simulink model "DoAero_2008a"  (Simulink 7.1)
settings: Solver=ode3  StartTime=0.0  StopTime=100  FixedStep=0.01  RelTol=1e-3
settings Model: Creator=abdelrazzak.merheb  LastModifiedBy=flying
settings OptimizationCC: InitFltsAndDblsToZero=off
settings DebuggingCC: StrictBusMsg=ErrorLevel1
settings CodeAppCC: CustomSymbolStrType=$N$R$M_T
settings GRTTargetCC: TargetFunctionLibrary=C89/C90 (ANSI)  CPPClassGenCompliant=off

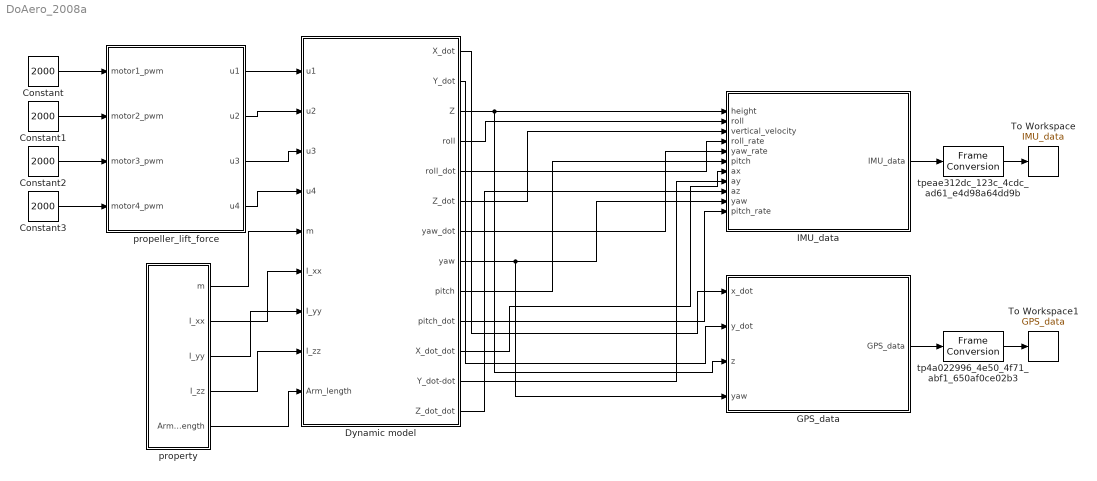
== system DoAero_2008a ==
  Constant{,1..3} (4 alike) : Constant  Value=2000
  Dynamic model : Subsystem
  GPS_data : Subsystem
  IMU_data : Subsystem
  To Workspace : ToWorkspace  VariableName=IMU_data  SampleTime=-1
  To Workspace1 : ToWorkspace  VariableName=GPS_data  SampleTime=-1
  propeller_lift_force : Stateflow chart  TreatAsAtomicUnit=on
      settings: PermitHierarchicalResolution=ParametersOnly
  "property " : Subsystem
  tp4a022996_4e50_4f71_abf1_650af0ce02b3 : FrameConversion
  tpeae312dc_123c_4cdc_ad61_e4d98a64dd9b : FrameConversion
  wires:
  Dynamic model/9(pitch) -> IMU_data/6(pitch)
  Dynamic model/3(Z) -> GPS_data/3(z), IMU_data/1(height)
  Dynamic model/4(roll) -> IMU_data/2(roll)
  Dynamic model/6(Z_dot) -> IMU_data/3(vertical_velocity)
  Dynamic model/5(roll_dot) -> IMU_data/4(roll_rate)
  Dynamic model/10(pitch_dot) -> IMU_data/11(pitch_rate)
  Dynamic model/7(yaw_dot) -> IMU_data/5(yaw_rate)
  Dynamic model/8(yaw) -> GPS_data/4(yaw), IMU_data/10(yaw)
  Dynamic model/11(X_dot_dot) -> IMU_data/7(ax)
  Dynamic model/12(Y_dot-dot) -> IMU_data/8(ay)
  Dynamic model/13(Z_dot_dot) -> IMU_data/9(az)
  "property "/5("Arm_length ") -> Dynamic model/9(Arm_length)
  "property "/4(I_zz) -> Dynamic model/8(I_zz)
  "property "/3(I_yy) -> Dynamic model/7(I_yy)
  "property "/2(I_xx) -> Dynamic model/6(I_xx)
  "property "/1(m) -> Dynamic model/5(m)
  propeller_lift_force/2(u2) -> Dynamic model/2(u2)
  propeller_lift_force/3(u3) -> Dynamic model/3(u3)
  propeller_lift_force/1(u1) -> Dynamic model/1(u1)
  propeller_lift_force/4(u4) -> Dynamic model/4(u4)
  Dynamic model/1("X_dot ") -> GPS_data/1(x_dot)
  Dynamic model/2(Y_dot) -> GPS_data/2(y_dot)
  Constant/1 -> propeller_lift_force/1(motor1_pwm)
  Constant1/1 -> propeller_lift_force/2(motor2_pwm)
  Constant2/1 -> propeller_lift_force/3(motor3_pwm)
  Constant3/1 -> propeller_lift_force/4(motor4_pwm)
  IMU_data/1(IMU_data) -> tpeae312dc_123c_4cdc_ad61_e4d98a64dd9b/1
  tpeae312dc_123c_4cdc_ad61_e4d98a64dd9b/1 -> To Workspace/1
  GPS_data/1(GPS_data) -> tp4a022996_4e50_4f71_abf1_650af0ce02b3/1
  tp4a022996_4e50_4f71_abf1_650af0ce02b3/1 -> To Workspace1/1

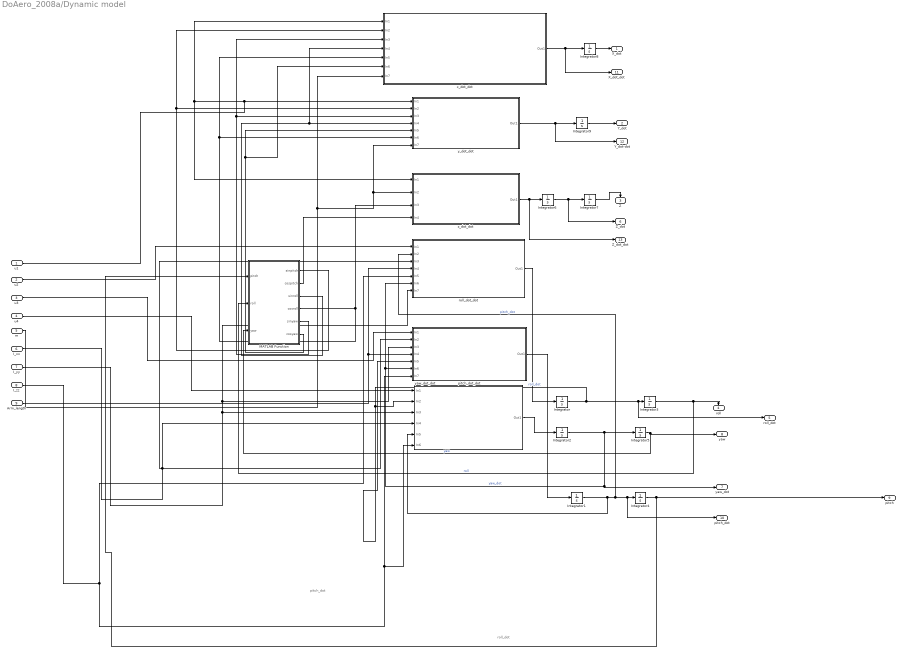
== system DoAero_2008a/Dynamic model ==
  note: pitch_dot
  note: roll_dot
  u1 : Inport
  u2 : Inport  Port=2
  u3 : Inport  Port=3
  u4 : Inport  Port=4
  m : Inport  Port=5
  I_xx : Inport  Port=6
  I_yy : Inport  Port=7
  I_zz : Inport  Port=8
  Arm_length : Inport  Port=9
  Integrator{,1..9} (10 alike) : Integrator
  MATLAB Function : Stateflow chart  TreatAsAtomicUnit=on
      settings: PermitHierarchicalResolution=ParametersOnly
  pitch_dot_dot : Subsystem
  roll_dot_dot : Subsystem
  x_dot_dot : Subsystem
  y_dot_dot : Subsystem
  yaw_dot_dot : Subsystem
  z_dot_dot : Subsystem
  "X_dot " : Outport
  Y_dot : Outport  Port=2
  Z : Outport  Orientation=down  Port=3
  roll : Outport  Orientation=down  Port=4
  roll_dot : Outport  Port=5
  Z_dot : Outport  Port=6
  yaw_dot : Outport  Port=7
  yaw : Outport  Port=8
  pitch : Outport  Port=9
  pitch_dot : Outport  Port=10
  X_dot_dot : Outport  Port=11
  Y_dot-dot : Outport  Port=12
  Z_dot_dot : Outport  Port=13
  wires:
  x_dot_dot/1(Out1) -> X_dot_dot/1, Integrator8/1
  Integrator6/1 -> Integrator7/1, Z_dot/1
  u4/1 -> yaw_dot_dot/1(In1)
  MATLAB Function/6(cosyaw) -> x_dot_dot/6(In6), y_dot_dot/5(In5)
  MATLAB Function/3(sinroll) -> x_dot_dot/4(In4), y_dot_dot/4(In4)
  MATLAB Function/4(cosroll) -> x_dot_dot/5(In5), y_dot_dot/6(In6), z_dot_dot/3(In3)
  MATLAB Function/1(sinpitch) -> x_dot_dot/2(In2), y_dot_dot/2(In2)
  m/1 -> x_dot_dot/7(In7), z_dot_dot/2(In2), y_dot_dot/7(In7)
  MATLAB Function/5(sinyaw) -> x_dot_dot/3(In3), y_dot_dot/3(In3)
  u1/1 -> y_dot_dot/1(In1), x_dot_dot/1(In1), z_dot_dot/1(In1)
  I_xx/1 -> yaw_dot_dot/4(In4), roll_dot_dot/3(In3), pitch_dot_dot/2(In2)
  I_yy/1 -> yaw_dot_dot/3(In3), roll_dot_dot/7(In7), pitch_dot_dot/3(In3)
  I_zz/1 -> roll_dot_dot/5(In5), yaw_dot_dot/6(In6), pitch_dot_dot/7(In7)
  Integrator3/1 -> roll/1, MATLAB Function/2(roll)  "roll"
  Integrator1/1 -> yaw_dot_dot/5(In5), roll_dot_dot/2(In2), pitch_dot/1, Integrator4/1  "pitch_dot"
  Integrator2/1 -> roll_dot_dot/6(In6), pitch_dot_dot/6(In6), yaw_dot/1, Integrator5/1  "yaw_dot"
  Integrator/1 -> pitch_dot_dot/5(In5), yaw_dot_dot/2(In2), roll_dot/1, Integrator3/1  "roll_dot"
  Integrator8/1 -> "X_dot "/1
  Integrator9/1 -> Y_dot/1
  Integrator5/1 -> MATLAB Function/3(yaw), yaw/1  "yaw"
  z_dot_dot/1(Out1) -> Z_dot_dot/1, Integrator6/1
  roll_dot_dot/1(Out1) -> Integrator/1
  pitch_dot_dot/1(Out1) -> Integrator1/1
  MATLAB Function/2(cospitch) -> z_dot_dot/4(In4)
  u2/1 -> roll_dot_dot/1(In1)
  Arm_length/1 -> roll_dot_dot/4(In4), pitch_dot_dot/4(In4)
  u3/1 -> pitch_dot_dot/1(In1)
  y_dot_dot/1(Out1) -> Y_dot-dot/1, Integrator9/1
  Integrator4/1 -> pitch/1, MATLAB Function/1(pitch)
  Integrator7/1 -> Z/1
  yaw_dot_dot/1(Out1) -> Integrator2/1

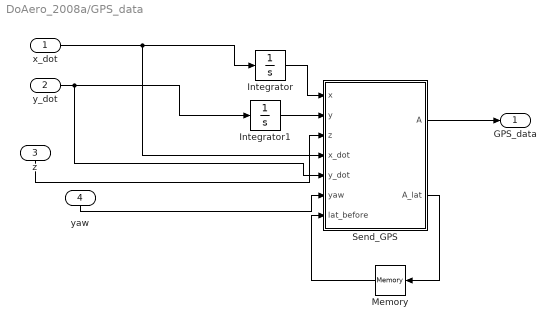
== system DoAero_2008a/GPS_data ==
  x_dot : Inport
  y_dot : Inport  Port=2
  z : Inport  Orientation=down  Port=3
  yaw : Inport  Orientation=down  Port=4
  Integrator : Integrator
  Integrator1 : Integrator
  Memory : Memory  Orientation=left  X0=30
  Send_GPS : Stateflow chart  TreatAsAtomicUnit=on
      settings: PermitHierarchicalResolution=ParametersOnly
  GPS_data : Outport
  wires:
  Integrator/1 -> Send_GPS/1(x)
  Integrator1/1 -> Send_GPS/2(y)
  Send_GPS/1(A) -> GPS_data/1
  yaw/1 -> Send_GPS/6(yaw)
  z/1 -> Send_GPS/3(z)
  Memory/1 -> Send_GPS/7(lat_before)
  Send_GPS/2(A_lat) -> Memory/1
  x_dot/1 -> Integrator/1, Send_GPS/4(x_dot)
  y_dot/1 -> Send_GPS/5(y_dot), Integrator1/1

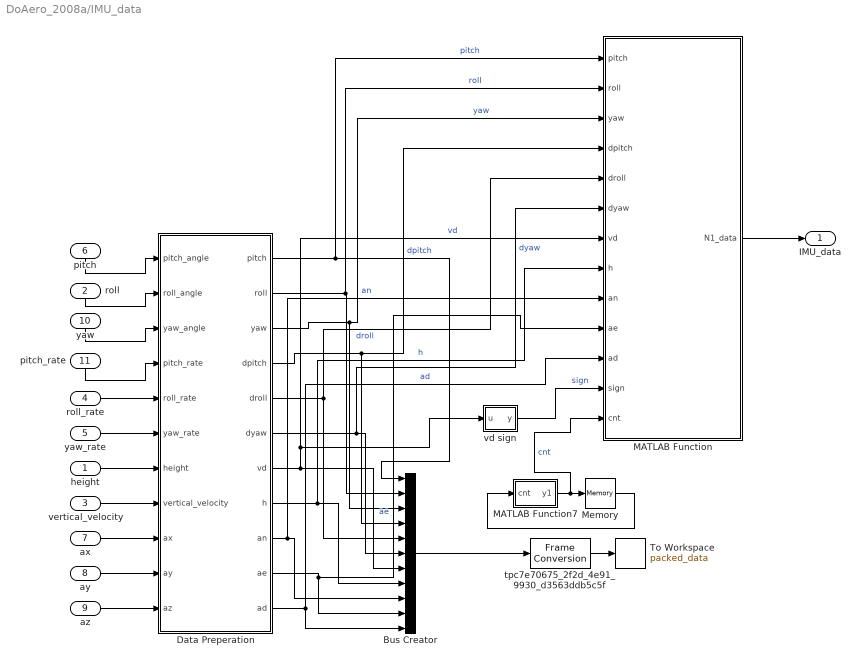
== system DoAero_2008a/IMU_data ==
  height : Inport
  roll : Inport  Orientation=down  Port=2
  vertical_velocity : Inport  Port=3
  roll_rate : Inport  Port=4
  yaw_rate : Inport  Port=5
  pitch : Inport  Orientation=down  Port=6
  ax : Inport  Port=7
  ay : Inport  Port=8
  az : Inport  Port=9
  yaw : Inport  Orientation=down  Port=10
  pitch_rate : Inport  Orientation=down  Port=11
  Bus Creator : BusCreator  Inputs=11
  Data Preperation : Stateflow chart  TreatAsAtomicUnit=on
      settings: PermitHierarchicalResolution=ParametersOnly
  MATLAB Function : Stateflow chart  TreatAsAtomicUnit=on
      settings: PermitHierarchicalResolution=ParametersOnly
  MATLAB Function7 : Stateflow chart  TreatAsAtomicUnit=on
      settings: PermitHierarchicalResolution=ParametersOnly
  Memory : Memory
  To Workspace : ToWorkspace  VariableName=packed_data  SampleTime=-1
  tpc7e70675_2f2d_4e91_9930_d3563ddb5c5f : FrameConversion
  vd sign : Stateflow chart  TreatAsAtomicUnit=on
      settings: PermitHierarchicalResolution=ParametersOnly
  IMU_data : Outport
  wires:
  Data Preperation/5(droll) -> MATLAB Function/5(droll), Bus Creator/5  "droll"
  Data Preperation/10(ae) -> MATLAB Function/10(ae), Bus Creator/10  "ae"
  ax/1 -> Data Preperation/9(ax)
  Data Preperation/6(dyaw) -> MATLAB Function/6(dyaw), Bus Creator/6  "dyaw"
  Data Preperation/7(vd) -> MATLAB Function/7(vd), vd sign/1(u), Bus Creator/7  "vd"
  Data Preperation/8(h) -> MATLAB Function/8(h), Bus Creator/8  "h"
  Data Preperation/3(yaw) -> MATLAB Function/3(yaw), Bus Creator/3  "yaw"
  Data Preperation/9(an) -> MATLAB Function/9(an), Bus Creator/9  "an"
  Data Preperation/4(dpitch) -> MATLAB Function/4(dpitch), Bus Creator/4  "dpitch"
  vd sign/1(y) -> MATLAB Function/12(sign)  "sign"
  MATLAB Function7/1(y1) -> MATLAB Function/13(cnt), Memory/1  "cnt"
  Data Preperation/2(roll) -> MATLAB Function/2(roll), Bus Creator/2  "roll"
  ay/1 -> Data Preperation/10(ay)
  Data Preperation/11(ad) -> MATLAB Function/11(ad), Bus Creator/11  "ad"
  Data Preperation/1(pitch) -> MATLAB Function/1(pitch), Bus Creator/1  "pitch"
  az/1 -> Data Preperation/11(az)
  Memory/1 -> MATLAB Function7/1(cnt)
  yaw_rate/1 -> Data Preperation/6(yaw_rate)
  height/1 -> Data Preperation/7(height)
  yaw/1 -> Data Preperation/3(yaw_angle)
  pitch/1 -> Data Preperation/1(pitch_angle)
  roll_rate/1 -> Data Preperation/5(roll_rate)
  pitch_rate/1 -> Data Preperation/4(pitch_rate)
  vertical_velocity/1 -> Data Preperation/8(vertical_velocity)
  roll/1 -> Data Preperation/2(roll_angle)
  MATLAB Function/1(N1_data) -> IMU_data/1
  Bus Creator/1 -> tpc7e70675_2f2d_4e91_9930_d3563ddb5c5f/1
  tpc7e70675_2f2d_4e91_9930_d3563ddb5c5f/1 -> To Workspace/1

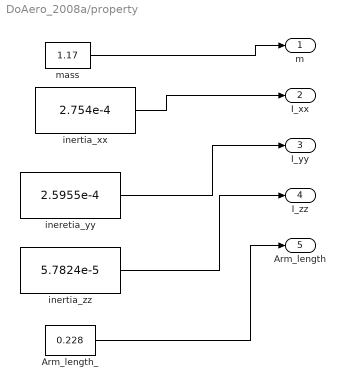
== system DoAero_2008a/property  ==
  Arm_length_ : Constant  Value=0.228
  ineretia_yy : Constant  Value=2.5955e-4
  inertia_xx : Constant  Value=2.754e-4
  inertia_zz : Constant  Value=5.7824e-5
  mass : Constant  Value=1.17
  m : Outport
  I_xx : Outport  Port=2
  I_yy : Outport  Port=3
  I_zz : Outport  Port=4
  "Arm_length " : Outport  Port=5
  wires:
  inertia_zz/1 -> I_zz/1
  Arm_length_/1 -> "Arm_length "/1
  ineretia_yy/1 -> I_yy/1
  mass/1 -> m/1
  inertia_xx/1 -> I_xx/1

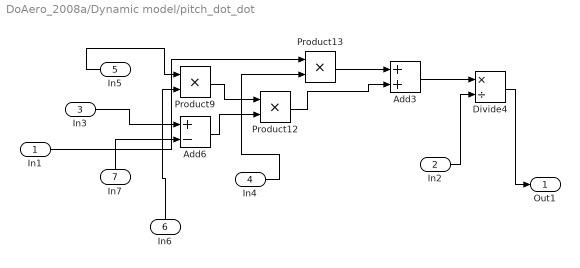
== system DoAero_2008a/Dynamic model/pitch_dot_dot ==
  In1 : Inport
  In2 : Inport  Port=2
  In3 : Inport  Port=3
  In4 : Inport  Port=4
  In5 : Inport  Orientation=left  Port=5
  In6 : Inport  Orientation=up  Port=6
  In7 : Inport  Orientation=up  Port=7
  Add3 : Sum
  Add6 : Sum  Inputs=+-
  Divide4 : Product  Inputs=*/
  Product12 : Product
  Product13 : Product
  Product9 : Product
  Out1 : Outport
  wires:
  Product12/1 -> Add3/2
  Product13/1 -> Add3/1
  In1/1 -> Product13/1
  Add6/1 -> Product12/2
  Add3/1 -> Divide4/1
  Product9/1 -> Product12/1
  In4/1 -> Product13/2
  In6/1 -> Product9/2
  In7/1 -> Add6/2
  In3/1 -> Add6/1
  In2/1 -> Divide4/2
  In5/1 -> Product9/1
  Divide4/1 -> Out1/1

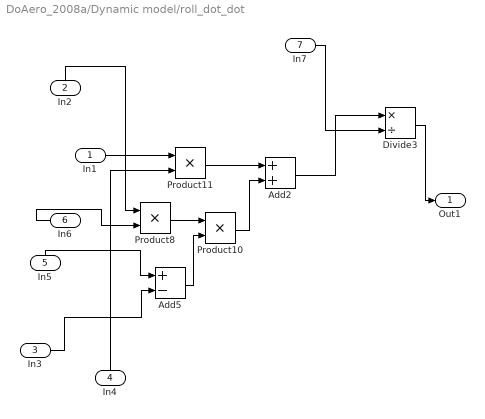
== system DoAero_2008a/Dynamic model/roll_dot_dot ==
  In1 : Inport
  In2 : Inport  Orientation=up  Port=2
  In3 : Inport  Port=3
  In4 : Inport  Orientation=up  Port=4
  In5 : Inport  Orientation=up  Port=5
  In6 : Inport  Orientation=left  Port=6
  In7 : Inport  Port=7
  Add2 : Sum
  Add5 : Sum  Inputs=+-
  Divide3 : Product  Inputs=*/
  Product10 : Product
  Product11 : Product
  Product8 : Product
  Out1 : Outport
  wires:
  Product11/1 -> Add2/1
  Add5/1 -> Product10/2
  In1/1 -> Product11/1
  Add2/1 -> Divide3/1
  Product8/1 -> Product10/1
  Product10/1 -> Add2/2
  Divide3/1 -> Out1/1
  In5/1 -> Add5/1
  In3/1 -> Add5/2
  In2/1 -> Product8/1
  In7/1 -> Divide3/2
  In4/1 -> Product11/2
  In6/1 -> Product8/2

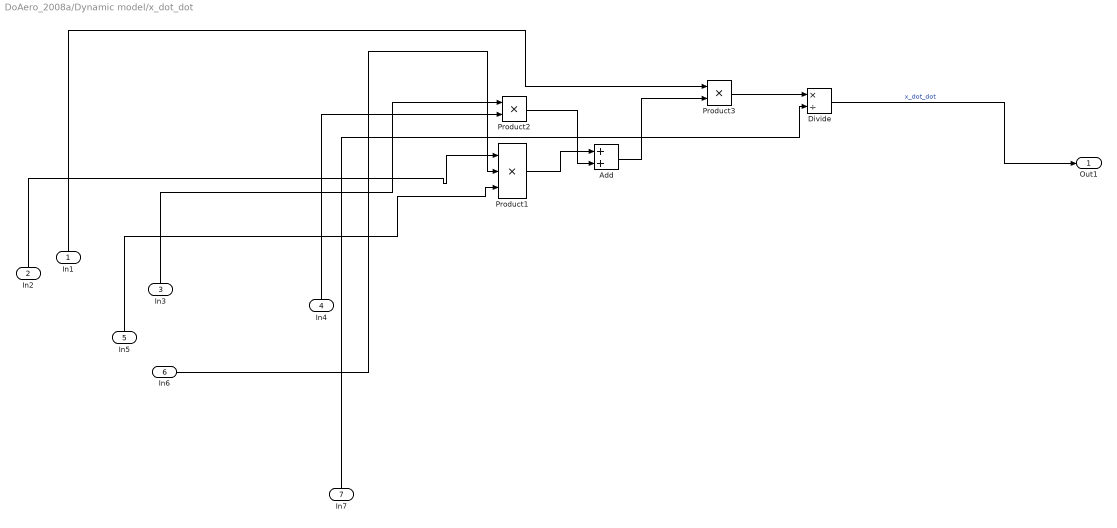
== system DoAero_2008a/Dynamic model/x_dot_dot ==
  In1 : Inport  Orientation=up
  In2 : Inport  Orientation=up  Port=2
  In3 : Inport  Orientation=up  Port=3
  In4 : Inport  Orientation=up  Port=4
  In5 : Inport  Orientation=up  Port=5
  In6 : Inport  Port=6
  In7 : Inport  Orientation=up  Port=7
  Add : Sum
  Divide : Product  Inputs=*/
  Product1 : Product  Inputs=3
  Product2 : Product
  Product3 : Product
  Out1 : Outport
  wires:
  In1/1 -> Product3/1
  In6/1 -> Product1/2
  In7/1 -> Divide/2
  In4/1 -> Product2/2
  In3/1 -> Product2/1
  In5/1 -> Product1/3
  In2/1 -> Product1/1
  Divide/1 -> Out1/1  "x_dot_dot"
  Product2/1 -> Add/2
  Product1/1 -> Add/1
  Product3/1 -> Divide/1
  Add/1 -> Product3/2

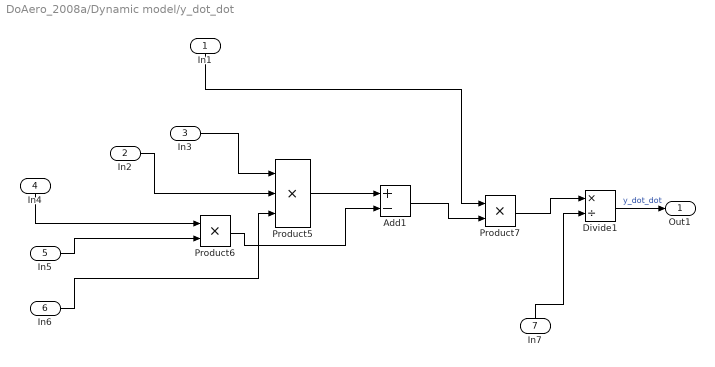
== system DoAero_2008a/Dynamic model/y_dot_dot ==
  In1 : Inport  Orientation=down
  In2 : Inport  Port=2
  In3 : Inport  Port=3
  In4 : Inport  Orientation=down  Port=4
  In5 : Inport  Port=5
  In6 : Inport  Port=6
  In7 : Inport  Orientation=up  Port=7
  Add1 : Sum  Inputs=+-
  Divide1 : Product  Inputs=*/
  Product5 : Product  Inputs=3
  Product6 : Product
  Product7 : Product
  Out1 : Outport
  wires:
  In1/1 -> Product7/1
  In2/1 -> Product5/2
  In5/1 -> Product6/2
  In7/1 -> Divide1/2
  In6/1 -> Product5/3
  In3/1 -> Product5/1
  In4/1 -> Product6/1
  Product5/1 -> Add1/1
  Add1/1 -> Product7/2
  Product6/1 -> Add1/2
  Divide1/1 -> Out1/1  "y_dot_dot"
  Product7/1 -> Divide1/1

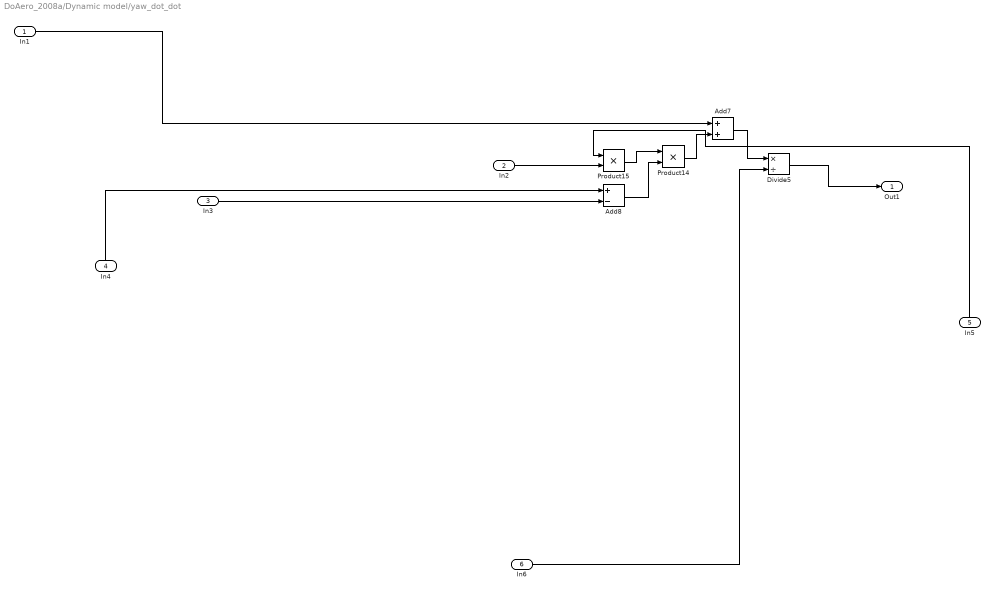
== system DoAero_2008a/Dynamic model/yaw_dot_dot ==
  In1 : Inport
  In2 : Inport  Port=2
  In3 : Inport  Port=3
  In4 : Inport  Orientation=up  Port=4
  In5 : Inport  Orientation=up  Port=5
  In6 : Inport  Port=6
  Add7 : Sum
  Add8 : Sum  Inputs=+-
  Divide5 : Product  Inputs=*/
  Product14 : Product
  Product15 : Product
  Out1 : Outport
  wires:
  In4/1 -> Add8/1
  In6/1 -> Divide5/2
  In2/1 -> Product15/2
  In3/1 -> Add8/2
  In5/1 -> Product15/1
  Product14/1 -> Add7/2
  Add8/1 -> Product14/2
  Product15/1 -> Product14/1
  In1/1 -> Add7/1
  Add7/1 -> Divide5/1
  Divide5/1 -> Out1/1

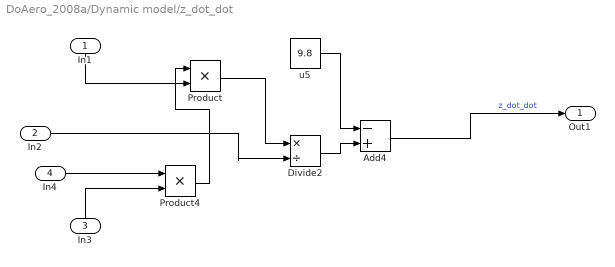
== system DoAero_2008a/Dynamic model/z_dot_dot ==
  In1 : Inport  Orientation=down
  In2 : Inport  Port=2
  In3 : Inport  Orientation=up  Port=3
  In4 : Inport  Port=4
  Add4 : Sum  Inputs=-+
  Divide2 : Product  Inputs=*/
  Product : Product
  Product4 : Product
  u5 : Constant  Value=9.8
  Out1 : Outport
  wires:
  In3/1 -> Product4/2
  In2/1 -> Divide2/2
  In1/1 -> Product/2
  Divide2/1 -> Add4/2
  Product4/1 -> Product/1
  In4/1 -> Product4/1
  u5/1 -> Add4/1
  Product/1 -> Divide2/1
  Add4/1 -> Out1/1  "z_dot_dot"

== matlab function IMU_data/vd sign ==
  data: u input double; y output double
function y = fcn(u)
if u>0;
y=bin2dec('00000000');
elseif u==0
y=bin2dec('00000000');
else u<0;
y=bin2dec('00000100');
end

== matlab function IMU_data/Data Preperation ==
  data: pitch output double; roll output double; yaw output double; pitch_angle input double; roll_angle input double; yaw_angle input double; pitch_rate input double; roll_rate input double; yaw_rate input double; dpitch output double; droll output double; dyaw output double; vd output double; h output double; height input double; an output double; ae output double; ad output double; vertical_velocity input double; ax input double; ay input double; az input double
function [pitch,roll,yaw,dpitch,droll,dyaw,vd,h,an,ae,ad] = fcn(pitch_angle,roll_angle,yaw_angle,pitch_rate,roll_rate,yaw_rate,height,vertical_velocity,ax,ay,az)

pitch=round(pitch_angle*573);
roll=round(roll_angle*573);
yaw=round(yaw_angle*573);


dpitch=round(pitch_rate*573);
droll=round(roll_rate*573);
dyaw=round(yaw_rate*573);


h=round(height*1000);
vd=round(vertical_velocity*100);


Rotation_metrix=[
                  cos(pitch_angle)*cos(yaw_angle)-cos(roll_angle)*sin(pitch_angle)*sin(yaw_angle),-cos(roll_angle)*cos(yaw_angle)*sin(pitch_angle)-cos(pitch_angle)*sin(yaw_angle),sin(pitch_angle)*sin(roll_angle);
                  cos(yaw_angle)*sin(pitch_angle)+cos(pitch_angle)*cos(roll_angle)*sin(yaw_angle),cos(pitch_angle)*cos(roll_angle)-sin(pitch_angle)*sin(yaw_angle),-cos(pitch_angle)*sin(roll_angle);
                  sin(roll_angle)*sin(yaw_angle),cos(yaw_angle)*sin(roll_angle),cos(roll_angle)
];

B=[ax,ay,az]';
A=Rotation_metrix*B;
an=A(1,1);
ae=A(2,1);
ad=A(3,1);

an=round(an*100);
ae=round(ae*100);
ad=round(ad*100);

== matlab function IMU_data/MATLAB Function ==
  data: pitch input double; N1_data output double; roll input double; yaw input double; dpitch input double; droll input double; dyaw input double; vd input double; h input double; an input double; ae input double; ad input double; sign input double; cnt input double
function N1_data= fcn(pitch,roll,yaw,dpitch,droll,dyaw,vd,h,an,ae,ad,sign,cnt)
%#eml

IMU_data_pack=zeros(1,41);

IMU_data_pack(1,1)=165;%帧头
IMU_data_pack(1,2)=90;%帧头
IMU_data_pack(1,3)=83;%帧长度
IMU_data_pack(1,4)=0;%保留
IMU_data_pack(1,5)=97;%帧标志
%数据段
IMU_data_pack(1,6)=127;%Flag0
IMU_data_pack(1,7)=11;%Flag1
IMU_data_pack(1,8)=128;%NavStatus
IMU_data_1_8=[IMU_data_pack(1,1),IMU_data_pack(1,2),IMU_data_pack(1,3),IMU_data_pack(1,4),IMU_data_pack(1,5),IMU_data_pack(1,6),    IMU_data_pack(1,7),IMU_data_pack(1,8)];

% Pitch,Roll,Yaw
IMU_data_pack(1,9)=pitch; %0,1
IMU_data_pack(1,10)=roll;%2,3
IMU_data_pack(1,11)=yaw;%4,5
IMU_data_9_10_11=[IMU_data_pack(1,9),IMU_data_pack(1,10),IMU_data_pack(1,11)];
%q0,q1,q2,q3
IMU_data_pack(1,12)=0;%6,7,8,9
IMU_data_pack(1,13)=0;%10,11,12,13
IMU_data_pack(1,14)=0;%14,15,16,17
IMU_data_pack(1,15)=0;%18,19,20,21
IMU_data_12_13_14_15=[IMU_data_pack(1,12),IMU_data_pack(1,13),IMU_data_pack(1,14),IMU_data_pack(1,15)];
%dpitch,droll,dyaw 22~27
IMU_data_pack(1,16)=dpitch;
IMU_data_pack(1,17)=droll;
IMU_data_pack(1,18)=dyaw;
IMU_data_9_10_11=[IMU_data_pack(1,16),IMU_data_pack(1,17),IMU_data_pack(1,18)];
%AngRateN,AngRateE,AngRateD 28~33
IMU_data_pack(1,19)=0;
IMU_data_pack(1,20)=0;
IMU_data_pack(1,21)=0;
IMU_data_19_20_21=[IMU_data_pack(1,19),IMU_data_pack(1,20),IMU_data_pack(1,21)];
%AngRateX,AngRateY,AngRateZ 34~39
IMU_data_pack(1,22)=0;
IMU_data_pack(1,23)=0;
IMU_data_pack(1,24)=0;
IMU_data_22_23_24=[IMU_data_pack(1,22),IMU_data_pack(1,23),IMU_data_pack(1,24)];
%Position 40~51
IMU_data_pack(1,25)=0;
IMU_data_pack(1,26)=0;
IMU_data_pack(1,27)=h;
IMU_data_25_26_27=[IMU_data_pack(1,25),IMU_data_pack(1,26),IMU_data_pack(1,27)];
%Velocity NED
IMU_data_pack(1,28)=sign;
%53~58
IMU_data_pack(1,29)=0;
IMU_data_pack(1,30)=0;
IMU_data_pack(1,31)=vd;
IMU_data_29_30_31=[IMU_data_pack(1,29),IMU_data_pack(1,30),IMU_data_pack(1,31)];
%Acceleration NED 59~64
IMU_data_pack(1,32)=an;
IMU_data_pack(1,33)=ae;
IMU_data_pack(1,34)=ad;
IMU_data_32_33_34=[IMU_data_pack(1,32),IMU_data_pack(1,33),IMU_data_pack(1,34)];
%Acceleration XYZ 65~70
IMU_data_pack(1,35)=0;
IMU_data_pack(1,36)=0;
IMU_data_pack(1,37)=0;
IMU_data_35_36_37=[IMU_data_pack(1,35),IMU_data_pack(1,36),IMU_data_pack(1,37)];
%AirHeight 71~74
IMU_data_pack(1,38)=h;
%cnt
IMU_data_pack(1,39)=cnt;

%%%%%%%%%%%%%Split Data for CRC 1~84
IMU_split_crc=zeros(1,87);
%1~8
j=1;
for i=1:1:8
IMU_split_crc(1,i)=IMU_data_pack(1,i);
j=j+1;
end
%9~14 pitch,roll,yaw
for i=9:1:11
    a=dec_to_bin_negative(IMU_data_pack(1,i),16);    
   IMU_split_crc(1,j)=bin2dec(a(9:16));
   j=j+1;
   IMU_split_crc(1,j)=bin2dec(a(1:8));
   j=j+1;
end
%15~30 q0,q1,q2,q3
for i=12:1:15
    a=dec_to_bin_negative(IMU_data_pack(1,i),32);
    IMU_split_crc(1,j)=bin2dec(a(25:32));
    j=j+1;
    IMU_split_crc(1,j)=bin2dec(a(17:24));
    j=j+1;
    IMU_split_crc(1,j)=bin2dec(a(9:16));
    j=j+1;
    IMU_split_crc(1,j)=bin2dec(a(1:8));
    j=j+1;
end
%31~36 dpitch,droll,dyaw
for i=16:1:18
a=dec_to_bin_negative(IMU_data_pack(1,i),16);
IMU_split_crc(1,j)=bin2dec(a(9:16));
j=j+1;
IMU_split_crc(1,j)=bin2dec(a(1:8));
j=j+1;
end
%37~42 AngRateN,AngRateE,AngRateD
for i=19:1:21
a=dec_to_bin_negative(IMU_data_pack(1,i),16);
IMU_split_crc(1,j)=bin2dec(a(9:16));
j=j+1;
IMU_split_crc(1,j)=bin2dec(a(1:8));
j=j+1;
end
%43~48 AngRateX,AngRateY,AngRateZ
for i=22:1:24
a=dec_to_bin_negative(IMU_data_pack(1,i),16);
IMU_split_crc(1,j)=bin2dec(a(9:16));
j=j+1;
IMU_split_crc(1,j)=bin2dec(a(1:8));
j=j+1;
end
%49~60 X,Y,Z
for i=25:1:27
a=dec_to_bin_negative(IMU_data_pack(1,i),32);
IMU_split_crc(1,j)=bin2dec(a(25:32));
j=j+1;
IMU_split_crc(1,j)=bin2dec(a(17:24));
j=j+1;
IMU_split_crc(1,j)=bin2dec(a(9:16));
j=j+1;
IMU_split_crc(1,j)=bin2dec(a(1:8));
j=j+1;
end
%61 sign
i=28;
a=dec_to_bin_negative(IMU_data_pack(1,i),8);
IMU_split_crc(1,j)=bin2dec(a(1:8));
j=j+1;
%62~67 VN,VE,VD 
for i=29:1:31
a=dec_to_bin_negative(IMU_data_pack(1,i),16);  
IMU_split_crc(1,j)=bin2dec(a(9:16));
j=j+1;
IMU_split_crc(1,j)=bin2dec(a(1:8));
j=j+1;
end
%68~73 an,ae,ad
for i=32:1:34
a=dec_to_bin_negative(IMU_data_pack(1,i),16);  
IMU_split_crc(1,j)=bin2dec(a(9:16));
j=j+1;
IMU_split_crc(1,j)=bin2dec(a(1:8));
j=j+1;
end
%74~79 ax,ay,az
for i=35:1:37
a=dec_to_bin_negative(IMU_data_pack(1,i),16);  
IMU_split_crc(1,j)=bin2dec(a(9:16));
j=j+1;
IMU_split_crc(1,j)=bin2dec(a(1:8));
j=j+1;
end
%80~83 height
i=38;
a=dec_to_bin_negative(IMU_data_pack(1,i),32);
IMU_split_crc(1,j)=bin2dec(a(25:32));
j=j+1;
IMU_split_crc(1,j)=bin2dec(a(17:24));
j=j+1;
IMU_split_crc(1,j)=bin2dec(a(9:16));
j=j+1;
IMU_split_crc(1,j)=bin2dec(a(1:8));
j=j+1;
%84 cnt
i=39;
a=dec_to_bin_negative(IMU_data_pack(1,i),8);
IMU_split_crc(1,j)=bin2dec(a(1:8));
%%%%%%%%%%%%%%%%%%%%%

%CRC
crc_gen=uint16(40961);
crc=uint16(65535);
buf_len=84;
 if (buf_len~=0)
    for i=1:1:buf_len
        crc=uint16(bitxor(crc,uint16(IMU_split_crc(1,i))));
        for j=1:1:8;           
        if (bitand(crc,1)==1)
           crc=uint16(bitshift(crc,-1));
           crc=uint16(bitxor(crc,crc_gen));
       else
           crc=uint16(bitshift(crc,-1));
       end
        end
    end
 end
IMU_data_pack(1,40)=crc;

a=dec_to_bin_negative(IMU_data_pack(1,40),16);
IMU_split_crc(1,85)=bin2dec(a(9:16));
IMU_split_crc(1,86)=bin2dec(a(1:8));


%checksum
checksum=0;
for j=1:1:86;     
   checksum=checksum+IMU_split_crc(1,j);     
end

checksum_bin=dec2bin(checksum,32);
checksum=bin2dec(checksum_bin(25:32));
IMU_split_crc(1,87)=checksum;

N1_data=IMU_split_crc;

== matlab function GPS_data/Send_GPS ==
  data: x input double; A output double; y input double; z input double; x_dot input double; y_dot input double; yaw input double; lat_before input double; A_lat output double
function [A,A_lat]= fcn(x,y,z,x_dot,y_dot,yaw,lat_before)

%GPGGA
A=zeros(1,36);
A(1,1)='$';
A(1,2)='G';
A(1,3)='P';
A(1,4)='G';
A(1,5)='G';
A(1,6)='A';
A(1,7)=2016;%UTC time <1>
A(1,8)=y/111318+30;%lat <2>
A_lat=A(1,8);
A(1,9)='N';%<3>
A(1,10)=x/110946/cos(lat_before*0.017453291)+120;%lon <4>
A(1,11)='E';%<5>
A(1,12)='0';%<6>
A(1,13)=12;%<7>
A(1,14)=0.5;%<8>
A(1,15)=z;%<9>
A(1,16)=z;%<10>
A(1,17)='*';


%GPRMC

A(1,18)='$';
A(1,19)='G';
A(1,20)='P';
A(1,21)='R';
A(1,22)='M';
A(1,23)='C';
A(1,24)=2016;%UTC time <1>
A(1,25)='A'; %<2>
A(1,26)=y/111318+30;  %<3>
A(1,27)='N';   %<4>
A(1,28)=x/110946/cos(lat_before*0.017453291)+120;  %<5>
A(1,29)='E'; %<6>
A(1,30)=sqrt(x_dot^2+y_dot^2);   %<7>
A(1,31)=yaw;%<8>
A(1,32)=2016;%<9>
A(1,33)=0;%<10>
A(1,34)='E';%<11>
A(1,35)='A';%<12>
A(1,36)='*';%<13>

== matlab function propeller_lift_force ==
  data: motor1_pwm input double; u1 output double; motor2_pwm input double; motor3_pwm input double; motor4_pwm input double; u2 output double; u3 output double; u4 output double
function [u1,u2,u3,u4] = fcn(motor1_pwm,motor2_pwm,motor3_pwm,motor4_pwm)

n1=(motor1_pwm-1050)*7.054+900;
n2=(motor2_pwm-1050)*7.054+900;
n3=(motor3_pwm-1050)*7.054+900;
n4=(motor4_pwm-1050)*7.054+900;


F1=1.0384e-7*n1^2;
F2=1.0384e-7*n2^2;
F3=1.0384e-7*n3^2;
F4=1.0384e-7*n4^2;

u1=F1+F2+F3+F4;
u2=F4-F2;
u3=F3-F1;
u4=F2+F4-F1-F3;

== matlab function Dynamic model/MATLAB Function ==
  data: pitch input double; sinpitch output double; roll input double; yaw input double; cospitch output double; sinroll output double; cosroll output double; sinyaw output double; cosyaw output double
function [sinpitch,cospitch,sinroll,cosroll,sinyaw,cosyaw]= fcn(pitch,roll,yaw)
sinpitch=sin(pitch);
cospitch=cos(pitch);
sinroll=sin(roll);
cosroll=cos(roll);
sinyaw=sin(yaw);
cosyaw=cos(yaw);

== matlab function IMU_data/MATLAB Function7 ==
  data: y1 output double; cnt input double
function y1= fcn(cnt)



y1=cnt+1;
if y1>255
y1=1;
end
